simulink model "NonlinearNoSlipPIDController_DAS_2016"  (R2018a)
settings: Solver=VariableStepAuto  StartTime=0.0  StopTime=100  MaxStep=0.1  RelTol=1e-8
InitFcn:
  | clearvars
  | 
  | % global t_change;
  | t_change=0;
  | 
  | T = 10;
  | a = 0.5;
  | b = 1;
  | v0 = 1;
  | 
  | % PID Gains
  | % kp = 10;
  | kp = 2*b/a^2;
  | TI = 5;
  | TD = 0.1;
  | 
  | % SM Gains
  | k0 = 20;
  | k1 = 0.05;
  | 
  | % DAS
  | DT=1;
  | gamma1sq=0.02;
  | gamma2sq=0.04;
  | % gamma1sq=0.2;
  | % gamma2sq=0.1;
  | y_ref=0;
libraries: simulink x2, vrlib x1, realtime_pacer_lib x1
settings Model: Creator=KvonEllenrieder  LastModifiedBy=transmogrifier
settings SolverCC: ZeroCrossAlgorithm=Adaptive
settings OptimizationCC: LifeSpan=inf
settings DebuggingCC: IgnoredZcDiagnostic=none  SFExecutionAtInitializationDiag=none
settings CodeAppCC: StateflowObjectComments=on

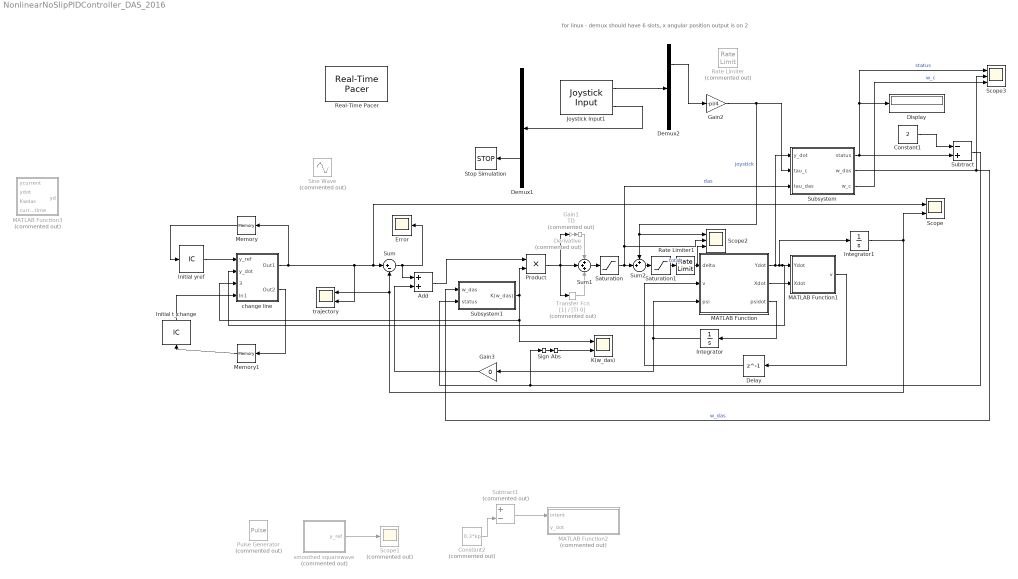
== system NonlinearNoSlipPIDController_DAS_2016 ==
  note: for linux - demux should have 6 slots, x angular position output is on 2
  Abs : Abs
  Add : Sum
  Constant1 : Constant  Value=2
  Constant2 : Constant  Commented=on  Value=0.3*kp
  Delay : Delay  DelayLength=1  InitialCondition=v0
  Demux1 : Demux  Outputs=10
  Demux2 : Demux  Outputs=6
  Derivative : Derivative  Commented=on
  Display : Display
  Error : Scope
  Gain1 : Gain  Commented=on  Gain=TD
  Gain2 : Gain  Gain=-pi/4
  Gain3 : Gain  Gain=0
  Initial t_change : InitialCondition  Value=0
  Initial yref : InitialCondition  Value=0
  Integrator : Integrator
  Integrator1 : Integrator
  Joystick Input1 : vrlib/Joystick Input  joyid=1  adjustports=on  forcefeed=off
      settings: SourceProductBaseCode=VR
  K(w_das) : Scope  NumInputPorts=2
  MATLAB Function : MATLAB Function  TreatAsAtomicUnit=on
  MATLAB Function1 : MATLAB Function  TreatAsAtomicUnit=on
  MATLAB Function2 : MATLAB Function  Commented=on  TreatAsAtomicUnit=on
  MATLAB Function3 : MATLAB Function  Commented=on  TreatAsAtomicUnit=on
  Memory : Memory
  Memory1 : Memory
  Product : Product
  Pulse Generator : DiscretePulseGenerator  Commented=on  PulseType=Time based  Amplitude=1.5  Period=T  PulseWidth=50
  Rate Limiter : RateLimiter  Commented=on  SampleTimeMode=inherited
  Rate Limiter1 : RateLimiter  RisingSlewLimit=0.5  FallingSlewLimit=-0.5  SampleTimeMode=inherited
  Real-Time Pacer : realtime_pacer_lib/Real-Time Pacer  simTimePerRealTime=1
  Saturation : Saturate  UpperLimit=pi/4  LowerLimit=-pi/4
  Saturation1 : Saturate  UpperLimit=pi/4  LowerLimit=-pi/4
  Scope : Scope  NumInputPorts=2
  Scope1 : Scope  Commented=on
  Scope2 : Scope  NumInputPorts=3
  Scope3 : Scope  NumInputPorts=3
  Sign : Signum
  Sine Wave : Sin  Commented=on  Amplitude=pi/4  Frequency=2*pi/T  SampleTime=0
  Stop Simulation : Stop
  Subsystem : Subsystem
  Subsystem1 : Subsystem
  Subtract : Sum  Inputs=-+
  Subtract1 : Sum  Commented=on  Inputs=+-
  Sum : Sum  Inputs=|+-
  Sum1 : Sum  Inputs=+++
  Sum2 : Sum  Inputs=++|
  Transfer Fcn : TransferFcn  Commented=on  Denominator=[TI 0]
  change line : Subsystem
  smoothed squarewave : Subsystem  Commented=on
  trajectory : Scope  NumInputPorts=2
  wires:
  MATLAB Function/3(psidot) -> Integrator/1
  Integrator/1 -> Gain3/1, MATLAB Function/3(psi)
  MATLAB Function/2(Xdot) -> MATLAB Function1/2(Xdot)
  MATLAB Function/1(Ydot) -> Subsystem/1(y_dot), Integrator1/1, change line/2(y_dot), MATLAB Function1/1(Ydot)
  MATLAB Function1/1(v) -> Delay/1
  Delay/1 -> MATLAB Function/2(v)
  Integrator1/1 -> Scope/2, Sum/2, trajectory/1
  change line/1(Out1) -> trajectory/2, Sum/1, Scope/1, Memory/1
  Saturation/1 -> Subsystem/3(tau_das), Scope2/2, Sum2/2  "das"
  Sum/1 -> Add/1, Error/1
  Sum1/1 -> Saturation/1
  Product/1 -> Gain1/1, Transfer Fcn/1, Sum1/2
  Transfer Fcn/1 -> Sum1/3
  Derivative/1 -> Sum1/1
  Gain1/1 -> Derivative/1
  smoothed squarewave/1(y_ref) -> Scope1/1
  Subsystem/1(status) -> Scope3/1, Display/1, Subtract/2  "status"
  Demux2/2 -> Gain2/1
  Joystick Input1/1 -> Demux2/1
  Joystick Input1/2 -> Demux1/1
  Demux1/8 -> Stop Simulation/1
  Sum2/1 -> Saturation1/1
  Saturation1/1 -> Rate Limiter1/1  "total"
  Constant1/1 -> Subtract/1
  Subtract/1 -> Sign/1, Subsystem1/2(status)
  Subsystem/2(w_das) -> Scope3/2, Subsystem1/1(w_das)  "w_das"
  Constant2/1 -> Subtract1/2
  Subtract1/1 -> MATLAB Function2/1(intent)
  Subsystem1/1(K(w_das)) -> Product/2, K(w_das)/1, change line/3(K(w_das))
  Gain2/1 -> Scope2/1, Sum2/1, Subsystem/2(tau_c)  "joystick"
  Add/1 -> Product/1
  Gain3/1 -> Add/2
  Memory/1 -> Initial yref/1
  Initial yref/1 -> change line/1(y_ref)
  change line/2(Out2) -> Memory1/1
  Memory1/1 -> Initial t_change/1
  Initial t_change/1 -> change line/4(In1)
  Subsystem/3(w_c) -> Scope3/3  "w_c"
  Sign/1 -> Abs/1
  Abs/1 -> K(w_das)/2
  Rate Limiter1/1 -> Scope2/3, MATLAB Function/1(delta)

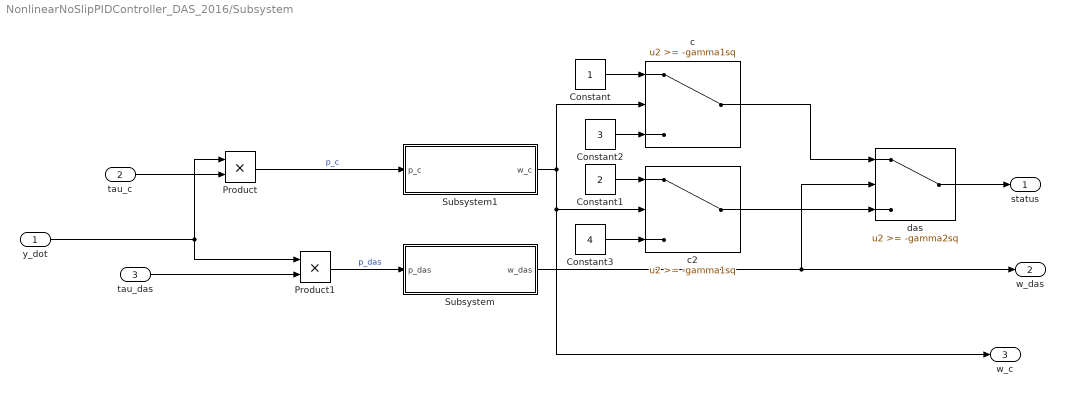
== system NonlinearNoSlipPIDController_DAS_2016/Subsystem ==
  y_dot : Inport
  tau_c : Inport  Port=2
  tau_das : Inport  Port=3
  Constant : Constant
  Constant1 : Constant  Value=2
  Constant2 : Constant  Value=3
  Constant3 : Constant  Value=4
  Product : Product
  Product1 : Product
  Subsystem : Subsystem
  Subsystem1 : Subsystem
  c : Switch  Threshold=-gamma1sq
  c2 : Switch  Threshold=-gamma1sq
  das : Switch  Threshold=-gamma2sq
  status : Outport
  w_das : Outport  Port=2
  w_c : Outport  Port=3
  wires:
  y_dot/1 -> Product/1, Product1/1
  tau_c/1 -> Product/2
  tau_das/1 -> Product1/2
  Product/1 -> Subsystem1/1(p_c)  "p_c"
  Product1/1 -> Subsystem/1(p_das)  "p_das"
  Subsystem/1(w_das) -> w_das/1, das/2
  Subsystem1/1(w_c) -> w_c/1, c2/2, c/2
  Constant/1 -> c/1
  c/1 -> das/1
  Constant1/1 -> c2/1
  c2/1 -> das/3
  Constant3/1 -> c2/3
  Constant2/1 -> c/3
  das/1 -> status/1

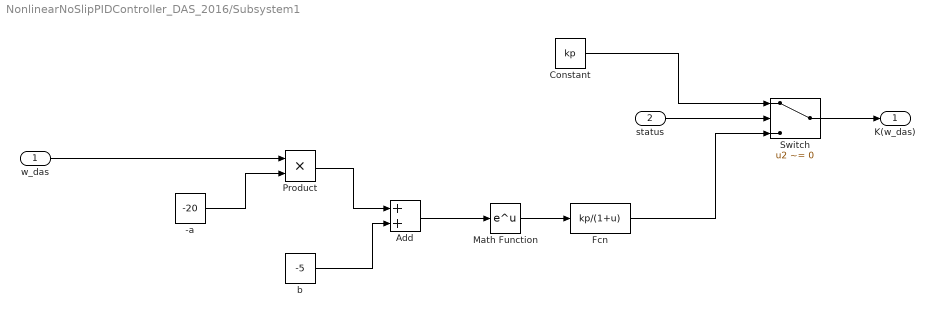
== system NonlinearNoSlipPIDController_DAS_2016/Subsystem1 ==
  w_das : Inport
  status : Inport  Port=2
  -a : Constant  Value=-20
  Add : Sum
  Constant : Constant  Value=kp
  Fcn : Fcn  Expr=kp/(1+u)
  Math Function : Math  SaturateOnIntegerOverflow=on
  Product : Product
  Switch : Switch  Criteria=u2 ~= 0
  b : Constant  Value=-5
  K(w_das) : Outport
  wires:
  w_das/1 -> Product/1
  -a/1 -> Product/2
  Product/1 -> Add/1
  b/1 -> Add/2
  Add/1 -> Math Function/1
  Math Function/1 -> Fcn/1
  Fcn/1 -> Switch/3
  status/1 -> Switch/2
  Switch/1 -> K(w_das)/1
  Constant/1 -> Switch/1

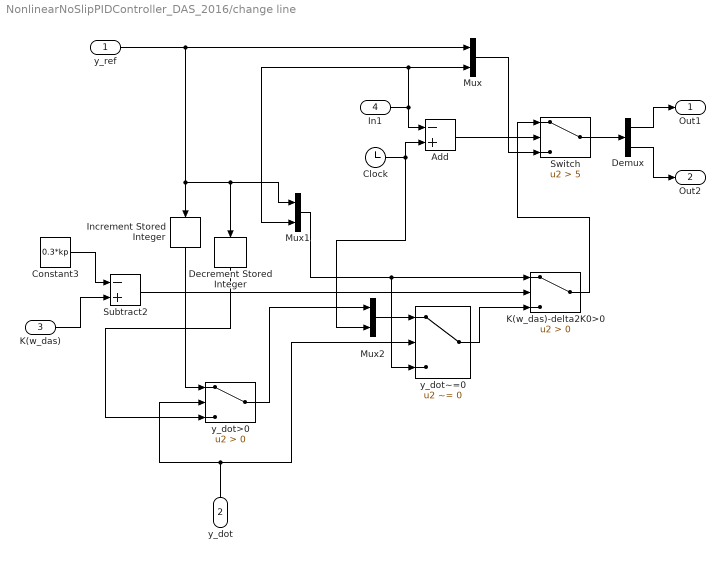
== system NonlinearNoSlipPIDController_DAS_2016/change line ==
  y_ref : Inport
  y_dot : Inport  Port=2
  K(w_das) : Inport  Port=3
  In1 : Inport  Port=4
  Add : Sum  Inputs=-+
  Clock : Clock
  Constant3 : Constant  Value=0.3*kp
  Decrement Stored Integer : simulink/Additional Math & Discrete/Additional Math: Increment - Decrement/Decrement Stored Integer
      settings: SourceProductName=Simulink  SourceProductBaseCode=SL
  Demux : Demux  Outputs=2
  Increment Stored Integer : simulink/Additional Math & Discrete/Additional Math: Increment - Decrement/Increment Stored Integer
      settings: SourceProductName=Simulink
  K(w_das)-delta2K0>0 : Switch  Criteria=u2 > Threshold  ZeroCross=off
  Mux : Mux  Inputs=2
  Mux1 : Mux  Inputs=2
  Mux2 : Mux  Inputs=2
  Subtract2 : Sum  Inputs=-+
  Switch : Switch  Criteria=u2 > Threshold  Threshold=5
  y_dot>0 : Switch  Criteria=u2 > Threshold
  y_dot~=0 : Switch  Criteria=u2 ~= 0
  Out1 : Outport
  Out2 : Outport  Port=2
  wires:
  Increment Stored Integer/1 -> y_dot>0/1
  Subtract2/1 -> K(w_das)-delta2K0>0/2
  y_dot>0/1 -> Mux2/1
  K(w_das)/1 -> Subtract2/2
  y_ref/1 -> Mux/1, Mux1/1, Decrement Stored Integer/1, Increment Stored Integer/1
  y_dot~=0/1 -> K(w_das)-delta2K0>0/3
  Constant3/1 -> Subtract2/1
  y_dot/1 -> y_dot~=0/2, y_dot>0/2
  Decrement Stored Integer/1 -> y_dot>0/3
  Clock/1 -> Mux2/2, Add/2
  In1/1 -> Add/1, Mux1/2, Mux/2
  Add/1 -> Switch/2
  K(w_das)-delta2K0>0/1 -> Switch/1
  Mux/1 -> Switch/3
  Switch/1 -> Demux/1
  Demux/1 -> Out1/1
  Demux/2 -> Out2/1
  Mux1/1 -> K(w_das)-delta2K0>0/1, y_dot~=0/3
  Mux2/1 -> y_dot~=0/1

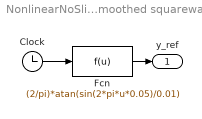
== system NonlinearNoSlipPIDController_DAS_2016/smoothed squarewave ==
  Clock : Clock
  Fcn : Fcn  Expr=(2/pi)*atan(sin(2*pi*u*0.05)/0.01)
  y_ref : Outport
  wires:
  Fcn/1 -> y_ref/1
  Clock/1 -> Fcn/1

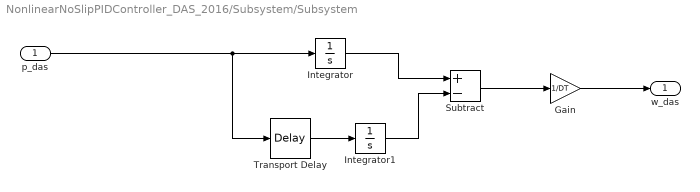
== system NonlinearNoSlipPIDController_DAS_2016/Subsystem/Subsystem ==
  p_das : Inport
  Gain : Gain  Gain=1/DT
  Integrator : Integrator
  Integrator1 : Integrator
  Subtract : Sum  Inputs=+-
  Transport Delay : TransportDelay  DelayTime=DT
  w_das : Outport
  wires:
  Subtract/1 -> Gain/1
  Gain/1 -> w_das/1
  Transport Delay/1 -> Integrator1/1
  Integrator1/1 -> Subtract/2
  Integrator/1 -> Subtract/1
  p_das/1 -> Transport Delay/1, Integrator/1

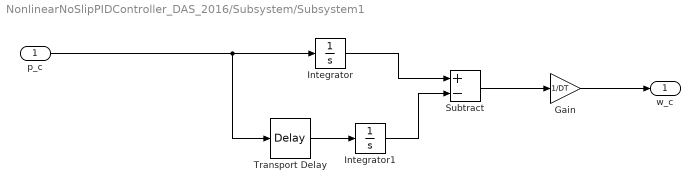
== system NonlinearNoSlipPIDController_DAS_2016/Subsystem/Subsystem1 ==
  p_c : Inport
  Gain : Gain  Gain=1/DT
  Integrator : Integrator
  Integrator1 : Integrator
  Subtract : Sum  Inputs=+-
  Transport Delay : TransportDelay  DelayTime=DT
  w_c : Outport
  wires:
  p_c/1 -> Integrator/1, Transport Delay/1
  Integrator/1 -> Subtract/1
  Integrator1/1 -> Subtract/2
  Transport Delay/1 -> Integrator1/1
  Gain/1 -> w_c/1
  Subtract/1 -> Gain/1

== matlab function NonlinearNoSlipPIDController_DAS_2016/MATLAB Function1 ==
  data: Ydot input; Xdot input; v output
function v = fcn(Ydot, Xdot)

v = sqrt(Xdot^2 + Ydot^2);

== matlab function NonlinearNoSlipPIDController_DAS_2016/MATLAB Function ==
  data: Ydot output; Xdot output; delta input; v input; psi input; a parameter; b parameter; psidot output; v0 parameter
function [Ydot, Xdot, psidot] = fcn(delta, v, psi, a, b, v0)

beta = atan(a*tan(delta)/b);

Xdot = v*cos(beta + psi);
Ydot = v*sin(beta + psi);

psidot = v0*tan(delta)/b;

== matlab function NonlinearNoSlipPIDController_DAS_2016/MATLAB Function2 ==
  data: intent input; y_dot input
function change_line(intent, y_dot)
coder.extrinsic('evalin', 'assignin')
y_ref=0;
y_ref = evalin('base','y_ref');
if intent < 0
    if y_dot < 0
        assignin('base','y_ref',y_ref-1);
    elseif y_dot > 0
        assignin('base','y_ref',y_ref+1);
    end
end
end

== matlab function NonlinearNoSlipPIDController_DAS_2016/MATLAB Function3 ==
  data: ycurrent input; yd output; ydot input; Kwdas input; kp parameter; current_time input
function yd = fcn(ycurrent, ydot, Kwdas, kp, current_time)
coder.extrinsic('evalin', 'assignin')

t_change=0;
t_change = evalin('base','t_change');

delta_sq = 0.3;

deltay = 1;

if Kwdas <= delta_sq*kp && current_time-t_change>0.5

    yd = ycurrent + sign(ydot)*deltay;
    % t_change=current_time;
    assignin('base','t_change',current_time);

else

    yd = ycurrent;

end
